simulink library "MedusaPremix"  (R2022b)
settings: Solver=VariableStepAuto  StartTime=0.0  StopTime=10.0  RelTol=1e-3
values from neighbouring files (symbols this model uses):
  PremixConfig = struct('sample_rate_in_hertz', sample_rate_in_hertz,                            'frame_size', frame_size,                            'rgain_SILENT_GAIN', rgain_SILENT_GAIN,                            'granularity', internal_granularity,                            'LR_in', LR_in, 'LR_out', LR_out,                            'CS_in', CS_in, 'CS_out', CS_out,                            'NumCenterOut' ...(+550 chars)    [MedusaPremixInit.m]
  PremixTune = MedusaPremixTuneInit(tuneFileName, headrestTuneFileName, overheadTuneFileName, MedusaParams)    [MedusaPremixInit.m]    (also in MedusaPremixTuneInit.m = load(tuneFileName))
undefined symbols (not defined in the file or in its folder): carModel, mode, MSConfig, Row
libraries: TuneVar x286, TOP x202, dspmtrx3 x146, FeaturePath x86, matrix_library x20, PooliirLib x8, Pooliir x4
(part 2 of 22)

== system MedusaPremix/Premix/Full Mixing Matrix_Center Surround ==
  Audio Channel Inputs : Inport
  RST Trigger : Inport  Port=2
  SLC Request Trigger : Inport  Port=3
  SLC In : Inport  Port=4
  SLC_NTF_check_done : Inport  Port=5
  SLC Tune In : Inport  Port=6
  Fade Request Trigger : Inport  Port=7
  Front Fade Gain : Inport  Port=8
  Back Fade Gain : Inport  Port=9
  Fade Tune In : Inport  Port=10
  Add : Sum
  Constant : Constant  OutDataTypeStr=single
  Fader Downmix : Subsystem
  FeaturePath : FeaturePath/FeaturePath  FeatureName=CS  IsGroup=off  GroupNumber=-1  DeclarePackages=off  PackageNames=mode,carModel  IsToolGroup=off  TriggerInit=[760 24 875 131]
      settings: SourceProductName=Bose Talaria
  Matrix Multiply : Product
  Premixing : Subsystem
  Subtract : Sum  Inputs=+-
  Surround Level Control : Subsystem
  Output : Outport  VectorParamsAs1DForOutWhenUnconnected=off
  SLC_NTF_done : Outport  Port=2  VectorParamsAs1DForOutWhenUnconnected=off
  wires:
  Front Fade Gain/1 -> Fader Downmix/1(Front Fade Gain)
  Add/1 -> Premixing/2(Target Gain)  "Premix Matrix"
  Premixing/1(Output) -> Output/1
  Fader Downmix/2(DownmixingMatrix) -> Add/2
  SLC Tune In/1 -> Surround Level Control/5(Tuned Inputs)
  RST Trigger/1 -> Surround Level Control/1(RST Trigger)
  Surround Level Control/2(Ramping Done) -> SLC_NTF_done/1
  Matrix Multiply/1 -> Add/1
  SLC In/1 -> Surround Level Control/3(Control Inputs)
  Fade Tune In/1 -> Fader Downmix/3(Tuned Inputs)
  Fader Downmix/1(Downmix) -> Subtract/2
  Audio Channel Inputs/1 -> Premixing/1(Audio Channel Inputs)
  SLC Request Trigger/1 -> Surround Level Control/2(SLC Request Trigger)
  SLC_NTF_check_done/1 -> Surround Level Control/4(Check Done)
  Fade Request Trigger/1 -> Fader Downmix/Trigger
  Back Fade Gain/1 -> Fader Downmix/2(Back Fade Gain)
  Constant/1 -> Subtract/1
  Subtract/1 -> Matrix Multiply/2  "No Downmix"
  Surround Level Control/1(Gain Out) -> Matrix Multiply/1

== system MedusaPremix/Premix/Full Mixing Matrix_Left ==
  Audio Channel Inputs : Inport
  RST Trigger : Inport  Port=2
  SLC Request Trigger : Inport  Port=3
  SLC In : Inport  Port=4
  SLC_NTF_check_done : Inport  Port=5
  SLC Tune In : Inport  Port=6
  Fade Request Trigger : Inport  Port=7
  Front Fade Gain : Inport  Port=8
  Back Fade Gain : Inport  Port=9
  Fade Tune In : Inport  Port=10
  Add : Sum
  Constant : Constant  OutDataTypeStr=single
  Fader Downmix : Subsystem
  FeaturePath : FeaturePath/FeaturePath  FeatureName=Left  IsGroup=off  GroupNumber=-1  DeclarePackages=off  PackageNames=mode,carModel  IsToolGroup=off  TriggerInit=[760 24 875 131]
      settings: SourceProductName=Bose Talaria
  Matrix Multiply : Product
  Premixing : Subsystem
  Subtract : Sum  Inputs=+-
  Surround Level Control : Subsystem
  Output : Outport  VectorParamsAs1DForOutWhenUnconnected=off
  SLC_NTF_done : Outport  Port=2  VectorParamsAs1DForOutWhenUnconnected=off
  wires:
  Surround Level Control/1(Gain Out) -> Matrix Multiply/1
  Front Fade Gain/1 -> Fader Downmix/1(Front Fade Gain)
  Add/1 -> Premixing/2(Target Gain)  "Premix Matrix"
  Premixing/1(Output) -> Output/1
  SLC Tune In/1 -> Surround Level Control/5(Tuned Inputs)
  Surround Level Control/2(Ramping Done) -> SLC_NTF_done/1
  Matrix Multiply/1 -> Add/1
  Fade Tune In/1 -> Fader Downmix/3(Tuned Inputs)
  Fader Downmix/1(Downmix) -> Subtract/2
  Audio Channel Inputs/1 -> Premixing/1(Audio Channel Inputs)
  SLC In/1 -> Surround Level Control/3(Control Inputs)
  SLC Request Trigger/1 -> Surround Level Control/2(SLC Request Trigger)
  SLC_NTF_check_done/1 -> Surround Level Control/4(Check Done)
  Back Fade Gain/1 -> Fader Downmix/2(Back Fade Gain)
  RST Trigger/1 -> Surround Level Control/1(RST Trigger)
  Fade Request Trigger/1 -> Fader Downmix/Trigger
  Fader Downmix/2(DownmixingMatrix) -> Add/2
  Subtract/1 -> Matrix Multiply/2  "No Downmix"
  Constant/1 -> Subtract/1

== system MedusaPremix/Premix/Full Mixing Matrix_Right ==
  Audio Channel Inputs : Inport
  RST Trigger : Inport  Port=2
  SLC Request Trigger : Inport  Port=3
  SLC In : Inport  Port=4
  SLC_NTF_check_done : Inport  Port=5
  SLC Tune In : Inport  Port=6
  Fade Request Trigger : Inport  Port=7
  Front Fade Gain : Inport  Port=8
  Back Fade Gain : Inport  Port=9
  Fade Tune In : Inport  Port=10
  Add : Sum
  Constant : Constant  OutDataTypeStr=single
  Fader Downmix : Subsystem
  FeaturePath : FeaturePath/FeaturePath  FeatureName=Right  IsGroup=off  GroupNumber=-1  DeclarePackages=off  PackageNames=mode,carModel  IsToolGroup=off  TriggerInit=[760 24 875 131]
      settings: SourceProductName=Bose Talaria
  Matrix Multiply : Product
  Premixing : Subsystem
  Subtract : Sum  Inputs=+-
  Surround Level Control : Subsystem
  Output : Outport  VectorParamsAs1DForOutWhenUnconnected=off
  SLC_NTF_done : Outport  Port=2  VectorParamsAs1DForOutWhenUnconnected=off
  wires:
  Front Fade Gain/1 -> Fader Downmix/1(Front Fade Gain)
  Add/1 -> Premixing/2(Target Gain)  "Premix Matrix"
  Premixing/1(Output) -> Output/1
  Fader Downmix/2(DownmixingMatrix) -> Add/2
  SLC Tune In/1 -> Surround Level Control/5(Tuned Inputs)
  RST Trigger/1 -> Surround Level Control/1(RST Trigger)
  Surround Level Control/2(Ramping Done) -> SLC_NTF_done/1
  Matrix Multiply/1 -> Add/1
  SLC In/1 -> Surround Level Control/3(Control Inputs)
  Fade Tune In/1 -> Fader Downmix/3(Tuned Inputs)
  Fader Downmix/1(Downmix) -> Subtract/2
  Audio Channel Inputs/1 -> Premixing/1(Audio Channel Inputs)
  SLC Request Trigger/1 -> Surround Level Control/2(SLC Request Trigger)
  SLC_NTF_check_done/1 -> Surround Level Control/4(Check Done)
  Fade Request Trigger/1 -> Fader Downmix/Trigger
  Back Fade Gain/1 -> Fader Downmix/2(Back Fade Gain)
  Constant/1 -> Subtract/1
  Subtract/1 -> Matrix Multiply/2  "No Downmix"
  Surround Level Control/1(Gain Out) -> Matrix Multiply/1

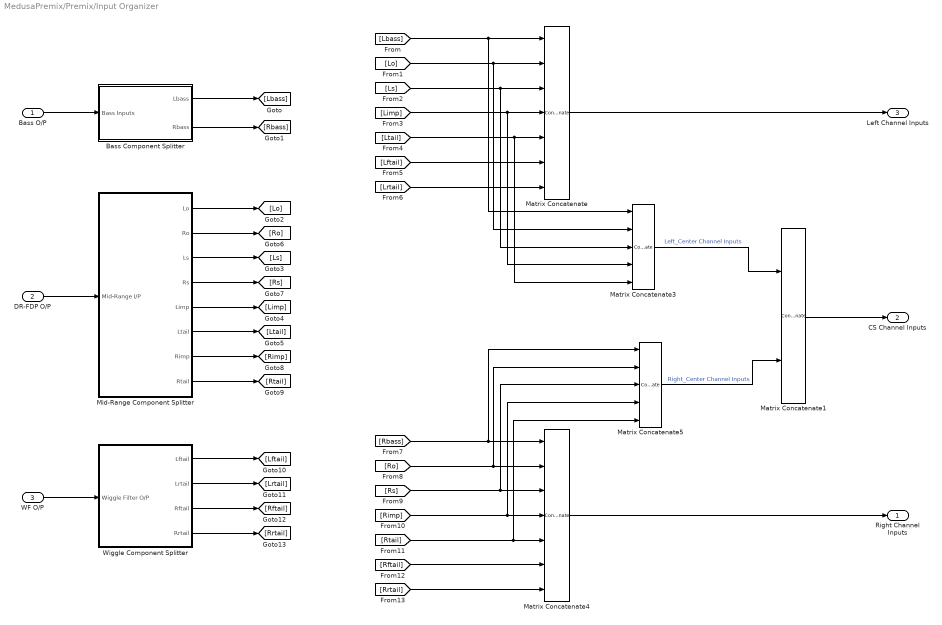
== system MedusaPremix/Premix/Input Organizer ==
  Bass O/P : Inport
  DR-FDP O/P : Inport  Port=2
  WF O/P : Inport  Port=3
  Bass Component Splitter : Subsystem
  Matrix Concatenate : Concatenate  NumInputs=7  Mode=Multidimensional array  ConcatenateDimension=2
  Matrix Concatenate1 : Concatenate  Mode=Multidimensional array  ConcatenateDimension=2
  Matrix Concatenate3 : Concatenate  NumInputs=5  Mode=Multidimensional array  ConcatenateDimension=2
  Matrix Concatenate4 : Concatenate  NumInputs=7  Mode=Multidimensional array  ConcatenateDimension=2
  Matrix Concatenate5 : Concatenate  NumInputs=5  Mode=Multidimensional array  ConcatenateDimension=2
  Mid-Range Component Splitter : Subsystem
  Wiggle Component Splitter : Subsystem
  Right Channel Inputs : Outport  VectorParamsAs1DForOutWhenUnconnected=off
  CS Channel Inputs : Outport  Port=2  VectorParamsAs1DForOutWhenUnconnected=off
  Left Channel Inputs : Outport  Port=3  VectorParamsAs1DForOutWhenUnconnected=off
  wires:
  Matrix Concatenate4/1 -> Right Channel Inputs/1
  [Ltail] -> Matrix Concatenate3/5, Matrix Concatenate/5
  Matrix Concatenate5/1 -> Matrix Concatenate1/2  "Right_Center Channel Inputs"
  [Limp] -> Matrix Concatenate3/4, Matrix Concatenate/4
  [Rimp] -> Matrix Concatenate5/4, Matrix Concatenate4/4
  [Rbass] -> Matrix Concatenate5/1, Matrix Concatenate4/1
  Matrix Concatenate1/1 -> CS Channel Inputs/1
  Wiggle Component Splitter/2(Lrtail) -> [Lrtail]
  Wiggle Component Splitter/1(Lftail) -> [Lftail]
  Bass Component Splitter/2(Rbass) -> [Rbass]
  DR-FDP O/P/1 -> Mid-Range Component Splitter/1(Mid-Range I/P)
  [Ro] -> Matrix Concatenate5/2, Matrix Concatenate4/2
  Wiggle Component Splitter/3(Rftail) -> [Rftail]
  Bass O/P/1 -> Bass Component Splitter/1(Bass Inputs)
  Matrix Concatenate/1 -> Left Channel Inputs/1
  [Lrtail] -> Matrix Concatenate/7
  [Lftail] -> Matrix Concatenate/6
  [Rs] -> Matrix Concatenate5/3, Matrix Concatenate4/3
  WF O/P/1 -> Wiggle Component Splitter/1(Wiggle Filter O/P)
  [Rtail] -> Matrix Concatenate5/5, Matrix Concatenate4/5
  [Ls] -> Matrix Concatenate3/3, Matrix Concatenate/3
  [Lbass] -> Matrix Concatenate3/1, Matrix Concatenate/1
  Matrix Concatenate3/1 -> Matrix Concatenate1/1  "Left_Center Channel Inputs"
  [Lo] -> Matrix Concatenate3/2, Matrix Concatenate/2
  Wiggle Component Splitter/4(Rrtail) -> [Rrtail]
  Mid-Range Component Splitter/1(Lo) -> [Lo]
  [Rftail] -> Matrix Concatenate4/6
  Bass Component Splitter/1(Lbass) -> [Lbass]
  [Rrtail] -> Matrix Concatenate4/7
  Mid-Range Component Splitter/2(Ro) -> [Ro]
  Mid-Range Component Splitter/3(Ls) -> [Ls]
  Mid-Range Component Splitter/4(Rs) -> [Rs]
  Mid-Range Component Splitter/5(Limp) -> [Limp]
  Mid-Range Component Splitter/6(Ltail) -> [Ltail]
  Mid-Range Component Splitter/7(Rimp) -> [Rimp]
  Mid-Range Component Splitter/8(Rtail) -> [Rtail]

== system MedusaPremix/Premix/Merge NTF_done ==
  SLC_NTF_done_Left : Inport
  SLC_NTF_done_CS : Inport  Port=2
  SLC_NTF_done_Right : Inport  Port=3
  Trigger : TriggerPort  TriggerType=function-call  VariantControl=Variant  PortDimensions=1
  AND : Logic  Inputs=3  IconShape=distinctive  AllPortsSameDT=off  OutDataTypeStr=boolean
  SLC_NTF_done : Outport  VectorParamsAs1DForOutWhenUnconnected=off
  wires:
  SLC_NTF_done_Right/1 -> AND/1
  SLC_NTF_done_CS/1 -> AND/2
  SLC_NTF_done_Left/1 -> AND/3
  AND/1 -> SLC_NTF_done/1

== system MedusaPremix/Premix/SLC Tuning ==
  Detent Level CS : Subsystem  Description="This is the premix (scalar mixing) matrix for the detent (default) level of \"surroundiness\"."
  Detent Level Left : Subsystem  Description="This is the premix (scalar mixing) matrix for the detent (default) level of \"surroundiness\"."
  Detent Level Right : Subsystem  Description="This is the premix (scalar mixing) matrix for the detent (default) level of \"surroundiness\"."
  Interpolation Method : Subsystem  Description=|
      | This controls the method used to interpolate premix coefficient matrix as the surround knob is adjusted.
      | - 0 for linear interpolation (default)
      | - 1 for db-linear interpolation
  Max Level CS : Subsystem  Description="This is the premix (scalar mixing) matrix for the maximum level of \"surroundiness\"."
  Max Level Left : Subsystem  Description="This is the premix (scalar mixing) matrix for the maximum level of \"surroundiness\"."
  Max Level Right : Subsystem  Description="This is the premix (scalar mixing) matrix for the maximum level of \"surroundiness\"."
  Min Level CS : Subsystem  Description="This is the premix (scalar mixing) matrix for the minimum level of \"surroundiness\" i.e. steroe case."
  Min Level Left : Subsystem  Description="This is the premix (scalar mixing) matrix for the minimum level of \"surroundiness\" i.e. steroe case."
  Min Level Right : Subsystem  Description="This is the premix (scalar mixing) matrix for the minimum level of \"surroundiness\" i.e. steroe case."
  Bus Element Out : Outport  VectorParamsAs1DForOutWhenUnconnected=off  PortName=SLC Tune Out  Element=Interpolation Method
  Bus Element Out1 : Outport  VectorParamsAs1DForOutWhenUnconnected=off  PortName=SLC Tune Out  Element=Min Level Left
  Bus Element Out2 : Outport  VectorParamsAs1DForOutWhenUnconnected=off  PortName=SLC Tune Out  Element=Detent Level Left
  Bus Element Out3 : Outport  VectorParamsAs1DForOutWhenUnconnected=off  PortName=SLC Tune Out  Element=Max Level Left
  Bus Element Out4 : Outport  VectorParamsAs1DForOutWhenUnconnected=off  PortName=SLC Tune Out  Element=Min Level CS
  Bus Element Out5 : Outport  VectorParamsAs1DForOutWhenUnconnected=off  PortName=SLC Tune Out  Element=Detent Level CS
  Bus Element Out6 : Outport  VectorParamsAs1DForOutWhenUnconnected=off  PortName=SLC Tune Out  Element=Max Level CS
  Bus Element Out7 : Outport  VectorParamsAs1DForOutWhenUnconnected=off  PortName=SLC Tune Out  Element=Min Level Right
  Bus Element Out8 : Outport  VectorParamsAs1DForOutWhenUnconnected=off  PortName=SLC Tune Out  Element=Detent Level Right
  Bus Element Out9 : Outport  VectorParamsAs1DForOutWhenUnconnected=off  PortName=SLC Tune Out  Element=Max Level Right
  wires:
  Interpolation Method/1(Out1) -> Bus Element Out/1
  Min Level Left/1(Out1) -> Bus Element Out1/1
  Detent Level Left/1(Out1) -> Bus Element Out2/1
  Max Level Left/1(Out1) -> Bus Element Out3/1
  Max Level CS/1(Out1) -> Bus Element Out6/1
  Min Level CS/1(Out1) -> Bus Element Out4/1
  Detent Level CS/1(Out1) -> Bus Element Out5/1
  Detent Level Right/1(Out1) -> Bus Element Out8/1
  Max Level Right/1(Out1) -> Bus Element Out9/1
  Min Level Right/1(Out1) -> Bus Element Out7/1

== system MedusaPremix/Premix51/Fade Inputs ==
  FrontGain : Inport
  BackGain : Inport  Port=2
  Abs : Abs  SaturateOnIntegerOverflow=off
  Abs1 : Abs  SaturateOnIntegerOverflow=off
  Add : Sum
  Delay : Delay  DelayLength=1  InitialCondition=0
  Delay1 : Delay  DelayLength=1  InitialCondition=0
  Fade_Trigger_Generation : MATLAB Function  TreatAsAtomicUnit=on
  Subtract1 : Sum  Inputs=-+
  Subtract2 : Sum  Inputs=-+
  triggerLeft : Outport  VectorParamsAs1DForOutWhenUnconnected=off
  triggerCS : Outport  Port=2  VectorParamsAs1DForOutWhenUnconnected=off
  triggerRight : Outport  Port=3  VectorParamsAs1DForOutWhenUnconnected=off
  FrontFadeGain : Outport  Port=4  VectorParamsAs1DForOutWhenUnconnected=off
  BackFadeGain : Outport  Port=5  VectorParamsAs1DForOutWhenUnconnected=off
  wires:
  Fade_Trigger_Generation/1(fadeTrigger_Left()) -> triggerLeft/1
  Fade_Trigger_Generation/3(fadeTrigger_Right()) -> triggerRight/1
  Add/1 -> Fade_Trigger_Generation/1(gainDifference)
  Fade_Trigger_Generation/2(fadeTrigger_CS()) -> triggerCS/1
  Delay1/1 -> Subtract2/1
  Delay/1 -> Subtract1/1
  FrontGain/1 -> Delay/1, FrontFadeGain/1, Subtract1/2
  Subtract1/1 -> Abs/1
  Subtract2/1 -> Abs1/1
  Abs/1 -> Add/1
  Abs1/1 -> Add/2
  BackGain/1 -> Delay1/1, Subtract2/2, BackFadeGain/1

== system MedusaPremix/Premix51/Fade Tuning ==
  Backward Downmix Max : Subsystem  Description=This is the fraction of downmixing that occurs when 100% fade (back) is reached.
  Backward Downmix Threshold : Subsystem  Description=This is the fraction of fade (back) at which downmixing of premix coefficients starts.
  Downmix Weights CS : Subsystem  Description=These are the mixing weights at fader extreme when downmix_max is set to 1.
  Downmix Weights Left : Subsystem  Description=These are the mixing weights at fader extreme when downmix_max is set to 1.
  Downmix Weights Right : Subsystem  Description=These are the mixing weights at fader extreme when downmix_max is set to 1.
  Forward Downmix Threshold : Subsystem  Description=This is the fraction of fade (front) at which downmixing of premix coefficients starts.
  Foward Downmix Max : Subsystem  Description=This is the fraction of downmixing that occurs when 100% fade (front) is reached.
  Bus Element Out : Outport  VectorParamsAs1DForOutWhenUnconnected=off  PortName=Fade Tune Out  Element=Forward Downmix Threshold
  Bus Element Out1 : Outport  VectorParamsAs1DForOutWhenUnconnected=off  PortName=Fade Tune Out  Element=Forward Downmix Max
  Bus Element Out2 : Outport  VectorParamsAs1DForOutWhenUnconnected=off  PortName=Fade Tune Out  Element=Backward Downmix Threshold
  Bus Element Out3 : Outport  VectorParamsAs1DForOutWhenUnconnected=off  PortName=Fade Tune Out  Element=Backward Downmix Max
  Bus Element Out4 : Outport  VectorParamsAs1DForOutWhenUnconnected=off  PortName=Fade Tune Out  Element=Downmix Weights Left
  Bus Element Out5 : Outport  VectorParamsAs1DForOutWhenUnconnected=off  PortName=Fade Tune Out  Element=Downmix Weights CS
  Bus Element Out6 : Outport  VectorParamsAs1DForOutWhenUnconnected=off  PortName=Fade Tune Out  Element=Downmix Weights Right
  wires:
  Forward Downmix Threshold/1(Out1) -> Bus Element Out/1
  Foward Downmix Max/1(Out1) -> Bus Element Out1/1
  Backward Downmix Max/1(Out1) -> Bus Element Out3/1
  Backward Downmix Threshold/1(Out1) -> Bus Element Out2/1
  Downmix Weights Left/1(Out1) -> Bus Element Out4/1
  Downmix Weights CS/1(Out1) -> Bus Element Out5/1
  Downmix Weights Right/1(Out1) -> Bus Element Out6/1

== system MedusaPremix/Premix51/Full Mixing Matrix_Center Surround ==
  Audio Channel Inputs : Inport
  RST Trigger : Inport  Port=2
  SLC Request Trigger : Inport  Port=3
  SLC In : Inport  Port=4
  SLC_NTF_check_done : Inport  Port=5
  SLC Tune In : Inport  Port=6
  Fade Request Trigger : Inport  Port=7
  Front Fade Gain : Inport  Port=8
  Back Fade Gain : Inport  Port=9
  Fade Tune In : Inport  Port=10
  Add : Sum
  Constant : Constant  OutDataTypeStr=single
  Fader Downmix : Subsystem
  FeaturePath : FeaturePath/FeaturePath  FeatureName=CS  IsGroup=off  GroupNumber=-1  DeclarePackages=off  PackageNames=mode,carModel  IsToolGroup=off  TriggerInit=[760 24 875 131]
      settings: SourceProductName=Bose Talaria
  Matrix Multiply : Product
  Premixing : Subsystem
  Subtract : Sum  Inputs=+-
  Surround Level Control : Subsystem
  Output : Outport  VectorParamsAs1DForOutWhenUnconnected=off
  SLC_NTF_done : Outport  Port=2  VectorParamsAs1DForOutWhenUnconnected=off
  wires:
  Surround Level Control/1(Gain Out) -> Matrix Multiply/1
  Front Fade Gain/1 -> Fader Downmix/1(Front Fade Gain)
  Add/1 -> Premixing/2(Target Gain)  "Premix Matrix"
  Premixing/1(Output) -> Output/1
  Fader Downmix/2(DownmixingMatrix) -> Add/2
  SLC Tune In/1 -> Surround Level Control/5(Tuned Inputs)
  RST Trigger/1 -> Surround Level Control/1(RST Trigger)
  Surround Level Control/2(Ramping Done) -> SLC_NTF_done/1
  Matrix Multiply/1 -> Add/1
  SLC In/1 -> Surround Level Control/3(Control Inputs)
  Fade Tune In/1 -> Fader Downmix/3(Tuned Inputs)
  Fader Downmix/1(Downmix) -> Subtract/2
  Audio Channel Inputs/1 -> Premixing/1(Audio Channel Inputs)
  SLC Request Trigger/1 -> Surround Level Control/2(SLC Request Trigger)
  SLC_NTF_check_done/1 -> Surround Level Control/4(Check Done)
  Fade Request Trigger/1 -> Fader Downmix/Trigger
  Back Fade Gain/1 -> Fader Downmix/2(Back Fade Gain)
  Constant/1 -> Subtract/1
  Subtract/1 -> Matrix Multiply/2  "No Downmix"

== system MedusaPremix/Premix51/Full Mixing Matrix_Left ==
  Audio Channel Inputs : Inport
  RST Trigger : Inport  Port=2
  SLC Request Trigger : Inport  Port=3
  SLC In : Inport  Port=4
  SLC_NTF_check_done : Inport  Port=5
  SLC Tune In : Inport  Port=6
  Fade Request Trigger : Inport  Port=7
  Front Fade Gain : Inport  Port=8
  Back Fade Gain : Inport  Port=9
  Fade Tune In : Inport  Port=10
  Add : Sum
  Constant : Constant  OutDataTypeStr=single
  Fader Downmix : Subsystem
  FeaturePath : FeaturePath/FeaturePath  FeatureName=Left  IsGroup=off  GroupNumber=-1  DeclarePackages=off  PackageNames=mode,carModel  IsToolGroup=off  TriggerInit=[760 24 875 131]
      settings: SourceProductName=Bose Talaria
  Matrix Multiply : Product
  Premixing : Subsystem
  Subtract : Sum  Inputs=+-
  Surround Level Control : Subsystem
  Output : Outport  VectorParamsAs1DForOutWhenUnconnected=off
  SLC_NTF_done : Outport  Port=2  VectorParamsAs1DForOutWhenUnconnected=off
  wires:
  Surround Level Control/1(Gain Out) -> Matrix Multiply/1
  Front Fade Gain/1 -> Fader Downmix/1(Front Fade Gain)
  Add/1 -> Premixing/2(Target Gain)  "Premix Matrix"
  Premixing/1(Output) -> Output/1
  SLC Tune In/1 -> Surround Level Control/5(Tuned Inputs)
  Surround Level Control/2(Ramping Done) -> SLC_NTF_done/1
  Matrix Multiply/1 -> Add/1
  Fade Tune In/1 -> Fader Downmix/3(Tuned Inputs)
  Fader Downmix/1(Downmix) -> Subtract/2
  Audio Channel Inputs/1 -> Premixing/1(Audio Channel Inputs)
  SLC In/1 -> Surround Level Control/3(Control Inputs)
  SLC Request Trigger/1 -> Surround Level Control/2(SLC Request Trigger)
  SLC_NTF_check_done/1 -> Surround Level Control/4(Check Done)
  Back Fade Gain/1 -> Fader Downmix/2(Back Fade Gain)
  RST Trigger/1 -> Surround Level Control/1(RST Trigger)
  Fade Request Trigger/1 -> Fader Downmix/Trigger
  Fader Downmix/2(DownmixingMatrix) -> Add/2
  Subtract/1 -> Matrix Multiply/2  "No Downmix"
  Constant/1 -> Subtract/1

== system MedusaPremix/Premix51/Full Mixing Matrix_Right ==
  Audio Channel Inputs : Inport
  RST Trigger : Inport  Port=2
  SLC Request Trigger : Inport  Port=3
  SLC In : Inport  Port=4
  SLC_NTF_check_done : Inport  Port=5
  SLC Tune In : Inport  Port=6
  Fade Request Trigger : Inport  Port=7
  Front Fade Gain : Inport  Port=8
  Back Fade Gain : Inport  Port=9
  Fade Tune In : Inport  Port=10
  Add : Sum
  Constant : Constant  OutDataTypeStr=single
  Fader Downmix : Subsystem
  FeaturePath : FeaturePath/FeaturePath  FeatureName=Right  IsGroup=off  GroupNumber=-1  DeclarePackages=off  PackageNames=mode,carModel  IsToolGroup=off  TriggerInit=[760 24 875 131]
      settings: SourceProductName=Bose Talaria
  Matrix Multiply : Product
  Premixing : Subsystem
  Subtract : Sum  Inputs=+-
  Surround Level Control : Subsystem
  Output : Outport  VectorParamsAs1DForOutWhenUnconnected=off
  SLC_NTF_done : Outport  Port=2  VectorParamsAs1DForOutWhenUnconnected=off
  wires:
  Surround Level Control/1(Gain Out) -> Matrix Multiply/1
  Front Fade Gain/1 -> Fader Downmix/1(Front Fade Gain)
  Add/1 -> Premixing/2(Target Gain)  "Premix Matrix"
  Premixing/1(Output) -> Output/1
  Fader Downmix/2(DownmixingMatrix) -> Add/2
  SLC Tune In/1 -> Surround Level Control/5(Tuned Inputs)
  RST Trigger/1 -> Surround Level Control/1(RST Trigger)
  Surround Level Control/2(Ramping Done) -> SLC_NTF_done/1
  Matrix Multiply/1 -> Add/1
  SLC In/1 -> Surround Level Control/3(Control Inputs)
  Fade Tune In/1 -> Fader Downmix/3(Tuned Inputs)
  Fader Downmix/1(Downmix) -> Subtract/2
  Audio Channel Inputs/1 -> Premixing/1(Audio Channel Inputs)
  SLC Request Trigger/1 -> Surround Level Control/2(SLC Request Trigger)
  SLC_NTF_check_done/1 -> Surround Level Control/4(Check Done)
  Fade Request Trigger/1 -> Fader Downmix/Trigger
  Back Fade Gain/1 -> Fader Downmix/2(Back Fade Gain)
  Constant/1 -> Subtract/1
  Subtract/1 -> Matrix Multiply/2  "No Downmix"

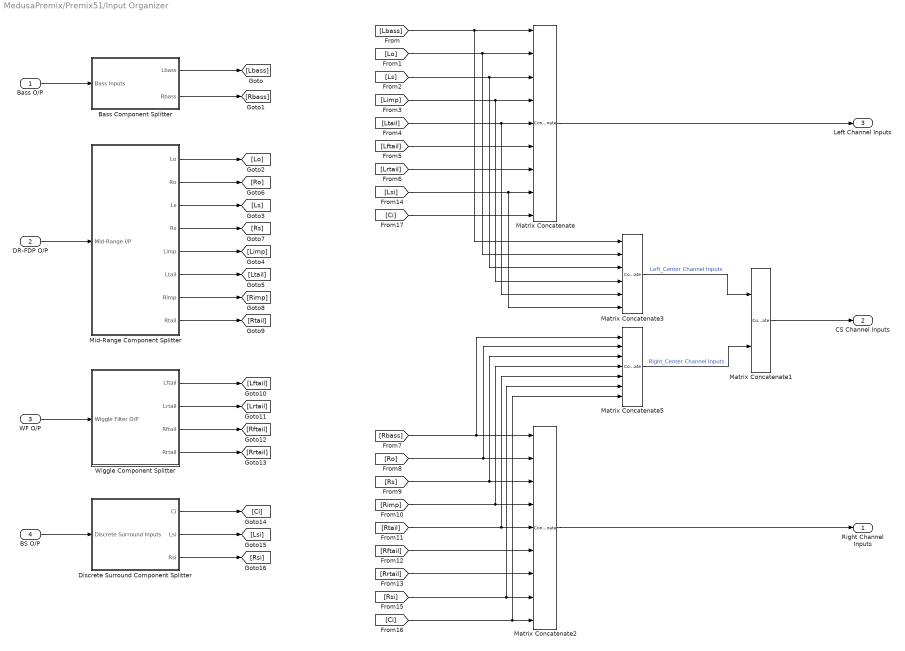
== system MedusaPremix/Premix51/Input Organizer ==
  Bass O/P : Inport
  DR-FDP O/P : Inport  Port=2
  WF O/P : Inport  Port=3
  BS O/P : Inport  Port=4
  Bass Component Splitter : Subsystem
  Discrete Surround Component Splitter : Subsystem
  Matrix Concatenate : Concatenate  NumInputs=9  Mode=Multidimensional array  ConcatenateDimension=2
  Matrix Concatenate1 : Concatenate  Mode=Multidimensional array  ConcatenateDimension=2
  Matrix Concatenate2 : Concatenate  NumInputs=9  Mode=Multidimensional array  ConcatenateDimension=2
  Matrix Concatenate3 : Concatenate  NumInputs=6  Mode=Multidimensional array  ConcatenateDimension=2
  Matrix Concatenate5 : Concatenate  NumInputs=7  Mode=Multidimensional array  ConcatenateDimension=2
  Mid-Range Component Splitter : Subsystem
  Wiggle Component Splitter : Subsystem
  Right Channel Inputs : Outport  VectorParamsAs1DForOutWhenUnconnected=off
  CS Channel Inputs : Outport  Port=2  VectorParamsAs1DForOutWhenUnconnected=off
  Left Channel Inputs : Outport  Port=3  VectorParamsAs1DForOutWhenUnconnected=off
  wires:
  Matrix Concatenate2/1 -> Right Channel Inputs/1
  [Ltail] -> Matrix Concatenate/5, Matrix Concatenate3/5
  Matrix Concatenate5/1 -> Matrix Concatenate1/2  "Right_Center Channel Inputs"
  [Limp] -> Matrix Concatenate/4, Matrix Concatenate3/4
  [Rimp] -> Matrix Concatenate2/4, Matrix Concatenate5/4
  [Rbass] -> Matrix Concatenate2/1, Matrix Concatenate5/1
  Matrix Concatenate1/1 -> CS Channel Inputs/1
  Wiggle Component Splitter/2(Lrtail) -> [Lrtail]
  Wiggle Component Splitter/1(Lftail) -> [Lftail]
  Bass Component Splitter/2(Rbass) -> [Rbass]
  DR-FDP O/P/1 -> Mid-Range Component Splitter/1(Mid-Range I/P)
  [Ro] -> Matrix Concatenate2/2, Matrix Concatenate5/2
  Wiggle Component Splitter/3(Rftail) -> [Rftail]
  Bass O/P/1 -> Bass Component Splitter/1(Bass Inputs)
  Matrix Concatenate/1 -> Left Channel Inputs/1
  [Lrtail] -> Matrix Concatenate/7
  [Lftail] -> Matrix Concatenate/6
  [Rs] -> Matrix Concatenate2/3, Matrix Concatenate5/3
  WF O/P/1 -> Wiggle Component Splitter/1(Wiggle Filter O/P)
  [Rtail] -> Matrix Concatenate2/5, Matrix Concatenate5/5
  [Ls] -> Matrix Concatenate/3, Matrix Concatenate3/3
  [Lbass] -> Matrix Concatenate/1, Matrix Concatenate3/1
  Matrix Concatenate3/1 -> Matrix Concatenate1/1  "Left_Center Channel Inputs"
  [Lo] -> Matrix Concatenate/2, Matrix Concatenate3/2
  Wiggle Component Splitter/4(Rrtail) -> [Rrtail]
  Mid-Range Component Splitter/1(Lo) -> [Lo]
  [Rftail] -> Matrix Concatenate2/6
  Bass Component Splitter/1(Lbass) -> [Lbass]
  [Rrtail] -> Matrix Concatenate2/7
  Mid-Range Component Splitter/2(Ro) -> [Ro]
  Mid-Range Component Splitter/3(Ls) -> [Ls]
  Mid-Range Component Splitter/4(Rs) -> [Rs]
  Mid-Range Component Splitter/5(Limp) -> [Limp]
  Mid-Range Component Splitter/6(Ltail) -> [Ltail]
  Mid-Range Component Splitter/7(Rimp) -> [Rimp]
  Mid-Range Component Splitter/8(Rtail) -> [Rtail]
  BS O/P/1 -> Discrete Surround Component Splitter/1(Discrete Surround Inputs)
  Discrete Surround Component Splitter/2(Lsi) -> [Lsi]
  Discrete Surround Component Splitter/1(Ci) -> [Ci]
  Discrete Surround Component Splitter/3(Rsi) -> [Rsi]
  [Lsi] -> Matrix Concatenate/8, Matrix Concatenate3/6
  [Rsi] -> Matrix Concatenate2/8, Matrix Concatenate5/6
  [Ci] -> Matrix Concatenate5/7, Matrix Concatenate2/9
  [Ci] -> Matrix Concatenate/9

== system MedusaPremix/Premix51/Merge NTF_done ==
  SLC_NTF_done_Left : Inport
  SLC_NTF_done_CS : Inport  Port=2
  SLC_NTF_done_Right : Inport  Port=3
  Trigger : TriggerPort  TriggerType=function-call  VariantControl=Variant  PortDimensions=1
  AND : Logic  Inputs=3  IconShape=distinctive  AllPortsSameDT=off  OutDataTypeStr=boolean
  SLC_NTF_done : Outport  VectorParamsAs1DForOutWhenUnconnected=off
  wires:
  SLC_NTF_done_Right/1 -> AND/1
  SLC_NTF_done_CS/1 -> AND/2
  SLC_NTF_done_Left/1 -> AND/3
  AND/1 -> SLC_NTF_done/1

== system MedusaPremix/Premix51/SLC Tuning ==
  Detent Level CS : Subsystem  Description="This is the premix (scalar mixing) matrix for the detent (default) level of \"surroundiness\"."
  Detent Level Left : Subsystem  Description="This is the premix (scalar mixing) matrix for the detent (default) level of \"surroundiness\"."
  Detent Level Right : Subsystem  Description="This is the premix (scalar mixing) matrix for the detent (default) level of \"surroundiness\"."
  Interpolation Method : Subsystem  Description=|
      | This controls the method used to interpolate premix coefficient matrix as the surround knob is adjusted.
      | - 0 for linear interpolation (default)
      | - 1 for db-linear interpolation
  Max Level CS : Subsystem  Description="This is the premix (scalar mixing) matrix for the maximum level of \"surroundiness\"."
  Max Level Left : Subsystem  Description="This is the premix (scalar mixing) matrix for the maximum level of \"surroundiness\"."
  Max Level Right : Subsystem  Description="This is the premix (scalar mixing) matrix for the maximum level of \"surroundiness\"."
  Min Level CS : Subsystem  Description="This is the premix (scalar mixing) matrix for the minimum level of \"surroundiness\" i.e. steroe case."
  Min Level Left : Subsystem  Description="This is the premix (scalar mixing) matrix for the minimum level of \"surroundiness\" i.e. steroe case."
  Min Level Right : Subsystem  Description="This is the premix (scalar mixing) matrix for the minimum level of \"surroundiness\" i.e. steroe case."
  Bus Element Out : Outport  VectorParamsAs1DForOutWhenUnconnected=off  PortName=SLC Tune Out  Element=Interpolation Method
  Bus Element Out1 : Outport  VectorParamsAs1DForOutWhenUnconnected=off  PortName=SLC Tune Out  Element=Min Level Left
  Bus Element Out2 : Outport  VectorParamsAs1DForOutWhenUnconnected=off  PortName=SLC Tune Out  Element=Detent Level Left
  Bus Element Out3 : Outport  VectorParamsAs1DForOutWhenUnconnected=off  PortName=SLC Tune Out  Element=Max Level Left
  Bus Element Out4 : Outport  VectorParamsAs1DForOutWhenUnconnected=off  PortName=SLC Tune Out  Element=Min Level CS
  Bus Element Out5 : Outport  VectorParamsAs1DForOutWhenUnconnected=off  PortName=SLC Tune Out  Element=Detent Level CS
  Bus Element Out6 : Outport  VectorParamsAs1DForOutWhenUnconnected=off  PortName=SLC Tune Out  Element=Max Level CS
  Bus Element Out7 : Outport  VectorParamsAs1DForOutWhenUnconnected=off  PortName=SLC Tune Out  Element=Min Level Right
  Bus Element Out8 : Outport  VectorParamsAs1DForOutWhenUnconnected=off  PortName=SLC Tune Out  Element=Detent Level Right
  Bus Element Out9 : Outport  VectorParamsAs1DForOutWhenUnconnected=off  PortName=SLC Tune Out  Element=Max Level Right
  wires:
  Interpolation Method/1(Out1) -> Bus Element Out/1
  Min Level Left/1(Out1) -> Bus Element Out1/1
  Detent Level Left/1(Out1) -> Bus Element Out2/1
  Max Level Left/1(Out1) -> Bus Element Out3/1
  Max Level CS/1(Out1) -> Bus Element Out6/1
  Min Level CS/1(Out1) -> Bus Element Out4/1
  Detent Level CS/1(Out1) -> Bus Element Out5/1
  Detent Level Right/1(Out1) -> Bus Element Out8/1
  Max Level Right/1(Out1) -> Bus Element Out9/1
  Min Level Right/1(Out1) -> Bus Element Out7/1

== system MedusaPremix/Premix51WithMonoSurround/CS Processing ==
  COut : Inport
  ChanIn : Inport  Port=2
  MixCoeff : Inport  Port=3
  Constant : Constant  Value=MedusaPremixConfig.NumSurroundOut  SampleTime=-1
  Mono-Surround : Subsystem
  Selective Concatenation : MATLAB Function  TreatAsAtomicUnit=on
  CSOut : Outport  VectorParamsAs1DForOutWhenUnconnected=off
  wires:
  ChanIn/1 -> Mono-Surround/1(ChanIn)
  Mono-Surround/1(S) -> Selective Concatenation/2(S)
  COut/1 -> Selective Concatenation/1(COut)
  MixCoeff/1 -> Mono-Surround/2(MixCoeff)
  Selective Concatenation/1(CSOut) -> CSOut/1
  Constant/1 -> Mono-Surround/Enable

== system MedusaPremix/Premix51WithMonoSurround/Fade Inputs ==
  FrontGain : Inport
  BackGain : Inport  Port=2
  Abs : Abs  SaturateOnIntegerOverflow=off
  Abs1 : Abs  SaturateOnIntegerOverflow=off
  Add : Sum
  Delay : Delay  DelayLength=1  InitialCondition=0
  Delay1 : Delay  DelayLength=1  InitialCondition=0
  Fade_Trigger_Generation : MATLAB Function  TreatAsAtomicUnit=on
  Subtract1 : Sum  Inputs=-+
  Subtract2 : Sum  Inputs=-+
  triggerLeft : Outport  VectorParamsAs1DForOutWhenUnconnected=off
  triggerCS : Outport  Port=2  VectorParamsAs1DForOutWhenUnconnected=off
  triggerRight : Outport  Port=3  VectorParamsAs1DForOutWhenUnconnected=off
  FrontFadeGain : Outport  Port=4  VectorParamsAs1DForOutWhenUnconnected=off
  BackFadeGain : Outport  Port=5  VectorParamsAs1DForOutWhenUnconnected=off
  wires:
  Fade_Trigger_Generation/1(fadeTrigger_Left()) -> triggerLeft/1
  Fade_Trigger_Generation/3(fadeTrigger_Right()) -> triggerRight/1
  Add/1 -> Fade_Trigger_Generation/1(gainDifference)
  Fade_Trigger_Generation/2(fadeTrigger_CS()) -> triggerCS/1
  Delay1/1 -> Subtract2/1
  Delay/1 -> Subtract1/1
  FrontGain/1 -> Delay/1, FrontFadeGain/1, Subtract1/2
  Subtract1/1 -> Abs/1
  Subtract2/1 -> Abs1/1
  Abs/1 -> Add/1
  Abs1/1 -> Add/2
  BackGain/1 -> Delay1/1, Subtract2/2, BackFadeGain/1

== system MedusaPremix/Premix51WithMonoSurround/Fade Tuning ==
  Backward Downmix Max : Subsystem  Description=This is the fraction of downmixing that occurs when 100% fade (back) is reached.
  Backward Downmix Threshold : Subsystem  Description=This is the fraction of fade (back) at which downmixing of premix coefficients starts.
  Downmix Weights CS : Subsystem  Description=These are the mixing weights at fader extreme when downmix_max is set to 1.
  Downmix Weights Left : Subsystem  Description=These are the mixing weights at fader extreme when downmix_max is set to 1.
  Downmix Weights Right : Subsystem  Description=These are the mixing weights at fader extreme when downmix_max is set to 1.
  Forward Downmix Threshold : Subsystem  Description=This is the fraction of fade (front) at which downmixing of premix coefficients starts.
  Foward Downmix Max : Subsystem  Description=This is the fraction of downmixing that occurs when 100% fade (front) is reached.
  Bus Element Out : Outport  VectorParamsAs1DForOutWhenUnconnected=off  PortName=Fade Tune Out  Element=Forward Downmix Threshold
  Bus Element Out1 : Outport  VectorParamsAs1DForOutWhenUnconnected=off  PortName=Fade Tune Out  Element=Forward Downmix Max
  Bus Element Out2 : Outport  VectorParamsAs1DForOutWhenUnconnected=off  PortName=Fade Tune Out  Element=Backward Downmix Threshold
  Bus Element Out3 : Outport  VectorParamsAs1DForOutWhenUnconnected=off  PortName=Fade Tune Out  Element=Backward Downmix Max
  Bus Element Out4 : Outport  VectorParamsAs1DForOutWhenUnconnected=off  PortName=Fade Tune Out  Element=Downmix Weights Left
  Bus Element Out5 : Outport  VectorParamsAs1DForOutWhenUnconnected=off  PortName=Fade Tune Out  Element=Downmix Weights CS
  Bus Element Out6 : Outport  VectorParamsAs1DForOutWhenUnconnected=off  PortName=Fade Tune Out  Element=Downmix Weights Right
  wires:
  Forward Downmix Threshold/1(Out1) -> Bus Element Out/1
  Foward Downmix Max/1(Out1) -> Bus Element Out1/1
  Backward Downmix Max/1(Out1) -> Bus Element Out3/1
  Backward Downmix Threshold/1(Out1) -> Bus Element Out2/1
  Downmix Weights Left/1(Out1) -> Bus Element Out4/1
  Downmix Weights CS/1(Out1) -> Bus Element Out5/1
  Downmix Weights Right/1(Out1) -> Bus Element Out6/1

== system MedusaPremix/Premix51WithMonoSurround/Full Mixing Matrix_Center Surround ==
  Audio Channel Inputs : Inport
  RST Trigger : Inport  Port=2
  SLC Request Trigger : Inport  Port=3
  SLC In : Inport  Port=4
  SLC_NTF_check_done : Inport  Port=5
  SLC Tune In : Inport  Port=6
  Fade Request Trigger : Inport  Port=7
  Front Fade Gain : Inport  Port=8
  Back Fade Gain : Inport  Port=9
  Fade Tune In : Inport  Port=10
  Add : Sum
  Constant : Constant  OutDataTypeStr=single
  Fader Downmix : Subsystem
  FeaturePath : FeaturePath/FeaturePath  FeatureName=CS  IsGroup=off  GroupNumber=-1  DeclarePackages=off  PackageNames=mode,carModel  IsToolGroup=off  TriggerInit=[760 24 875 131]
      settings: SourceProductName=Bose Talaria
  Matrix Multiply : Product
  Premixing : Subsystem
  Submatrix : dspmtrx3/Submatrix  RowSpan=One row  RowStartMode=Last  RowStartIndex=1  RowEndMode=Last  RowEndIndex=1  ColSpan=All columns  ColStartMode=First  ColStartIndex=1  ColEndMode=Last  ColEndIndex=1
  Submatrix1 : dspmtrx3/Submatrix  RowSpan=Range of rows  RowStartMode=First  RowStartIndex=1  RowEndMode=Index  RowEndIndex=MedusaPremixConfig.NumCenterOut  ColSpan=All columns  ColStartMode=First  ColStartIndex=1  ColEndMode=Last  ColEndIndex=1
  Subtract : Sum  Inputs=+-
  Surround Level Control : Subsystem
  Output : Outport  VectorParamsAs1DForOutWhenUnconnected=off
  MS Mixing Gains : Outport  Port=2  VectorParamsAs1DForOutWhenUnconnected=off
  SLC_NTF_done : Outport  Port=3  VectorParamsAs1DForOutWhenUnconnected=off
  wires:
  Surround Level Control/1(Gain Out) -> Matrix Multiply/1
  Front Fade Gain/1 -> Fader Downmix/1(Front Fade Gain)
  Premixing/1(Output) -> Output/1
  Fader Downmix/2(DownmixingMatrix) -> Add/2
  SLC Tune In/1 -> Surround Level Control/5(Tuned Inputs)
  RST Trigger/1 -> Surround Level Control/1(RST Trigger)
  Surround Level Control/2(Ramping Done) -> SLC_NTF_done/1
  Matrix Multiply/1 -> Add/1
  SLC In/1 -> Surround Level Control/3(Control Inputs)
  Fade Tune In/1 -> Fader Downmix/3(Tuned Inputs)
  Fader Downmix/1(Downmix) -> Subtract/2
  Audio Channel Inputs/1 -> Premixing/1(Audio Channel Inputs)
  SLC Request Trigger/1 -> Surround Level Control/2(SLC Request Trigger)
  SLC_NTF_check_done/1 -> Surround Level Control/4(Check Done)
  Fade Request Trigger/1 -> Fader Downmix/Trigger
  Back Fade Gain/1 -> Fader Downmix/2(Back Fade Gain)
  Constant/1 -> Subtract/1
  Subtract/1 -> Matrix Multiply/2  "No Downmix"
  Submatrix/1 -> MS Mixing Gains/1
  Add/1 -> Submatrix1/1, Submatrix/1  "Premix Matrix"
  Submatrix1/1 -> Premixing/2(Target Gain)

== system MedusaPremix/Premix51WithMonoSurround/Full Mixing Matrix_Left ==
  Audio Channel Inputs : Inport
  RST Trigger : Inport  Port=2
  SLC Request Trigger : Inport  Port=3
  SLC In : Inport  Port=4
  SLC_NTF_check_done : Inport  Port=5
  SLC Tune In : Inport  Port=6
  Fade Request Trigger : Inport  Port=7
  Front Fade Gain : Inport  Port=8
  Back Fade Gain : Inport  Port=9
  Fade Tune In : Inport  Port=10
  Add : Sum
  Constant : Constant  OutDataTypeStr=single
  Fader Downmix : Subsystem
  FeaturePath : FeaturePath/FeaturePath  FeatureName=Left  IsGroup=off  GroupNumber=-1  DeclarePackages=off  PackageNames=mode,carModel  IsToolGroup=off  TriggerInit=[760 24 875 131]
      settings: SourceProductName=Bose Talaria
  Matrix Multiply : Product
  Premixing : Subsystem
  Subtract : Sum  Inputs=+-
  Surround Level Control : Subsystem
  Output : Outport  VectorParamsAs1DForOutWhenUnconnected=off
  SLC_NTF_done : Outport  Port=2  VectorParamsAs1DForOutWhenUnconnected=off
  wires:
  Surround Level Control/1(Gain Out) -> Matrix Multiply/1
  Front Fade Gain/1 -> Fader Downmix/1(Front Fade Gain)
  Add/1 -> Premixing/2(Target Gain)  "Premix Matrix"
  Premixing/1(Output) -> Output/1
  SLC Tune In/1 -> Surround Level Control/5(Tuned Inputs)
  Surround Level Control/2(Ramping Done) -> SLC_NTF_done/1
  Matrix Multiply/1 -> Add/1
  Fade Tune In/1 -> Fader Downmix/3(Tuned Inputs)
  Fader Downmix/1(Downmix) -> Subtract/2
  Audio Channel Inputs/1 -> Premixing/1(Audio Channel Inputs)
  SLC In/1 -> Surround Level Control/3(Control Inputs)
  SLC Request Trigger/1 -> Surround Level Control/2(SLC Request Trigger)
  SLC_NTF_check_done/1 -> Surround Level Control/4(Check Done)
  Back Fade Gain/1 -> Fader Downmix/2(Back Fade Gain)
  RST Trigger/1 -> Surround Level Control/1(RST Trigger)
  Fade Request Trigger/1 -> Fader Downmix/Trigger
  Fader Downmix/2(DownmixingMatrix) -> Add/2
  Subtract/1 -> Matrix Multiply/2  "No Downmix"
  Constant/1 -> Subtract/1

== system MedusaPremix/Premix51WithMonoSurround/Full Mixing Matrix_Right ==
  Audio Channel Inputs : Inport
  RST Trigger : Inport  Port=2
  SLC Request Trigger : Inport  Port=3
  SLC In : Inport  Port=4
  SLC_NTF_check_done : Inport  Port=5
  SLC Tune In : Inport  Port=6
  Fade Request Trigger : Inport  Port=7
  Front Fade Gain : Inport  Port=8
  Back Fade Gain : Inport  Port=9
  Fade Tune In : Inport  Port=10
  Add : Sum
  Constant : Constant  OutDataTypeStr=single
  Fader Downmix : Subsystem
  FeaturePath : FeaturePath/FeaturePath  FeatureName=Right  IsGroup=off  GroupNumber=-1  DeclarePackages=off  PackageNames=mode,carModel  IsToolGroup=off  TriggerInit=[760 24 875 131]
      settings: SourceProductName=Bose Talaria
  Matrix Multiply : Product
  Premixing : Subsystem
  Subtract : Sum  Inputs=+-
  Surround Level Control : Subsystem
  Output : Outport  VectorParamsAs1DForOutWhenUnconnected=off
  SLC_NTF_done : Outport  Port=2  VectorParamsAs1DForOutWhenUnconnected=off
  wires:
  Surround Level Control/1(Gain Out) -> Matrix Multiply/1
  Front Fade Gain/1 -> Fader Downmix/1(Front Fade Gain)
  Add/1 -> Premixing/2(Target Gain)  "Premix Matrix"
  Premixing/1(Output) -> Output/1
  Fader Downmix/2(DownmixingMatrix) -> Add/2
  SLC Tune In/1 -> Surround Level Control/5(Tuned Inputs)
  RST Trigger/1 -> Surround Level Control/1(RST Trigger)
  Surround Level Control/2(Ramping Done) -> SLC_NTF_done/1
  Matrix Multiply/1 -> Add/1
  SLC In/1 -> Surround Level Control/3(Control Inputs)
  Fade Tune In/1 -> Fader Downmix/3(Tuned Inputs)
  Fader Downmix/1(Downmix) -> Subtract/2
  Audio Channel Inputs/1 -> Premixing/1(Audio Channel Inputs)
  SLC Request Trigger/1 -> Surround Level Control/2(SLC Request Trigger)
  SLC_NTF_check_done/1 -> Surround Level Control/4(Check Done)
  Fade Request Trigger/1 -> Fader Downmix/Trigger
  Back Fade Gain/1 -> Fader Downmix/2(Back Fade Gain)
  Constant/1 -> Subtract/1
  Subtract/1 -> Matrix Multiply/2  "No Downmix"

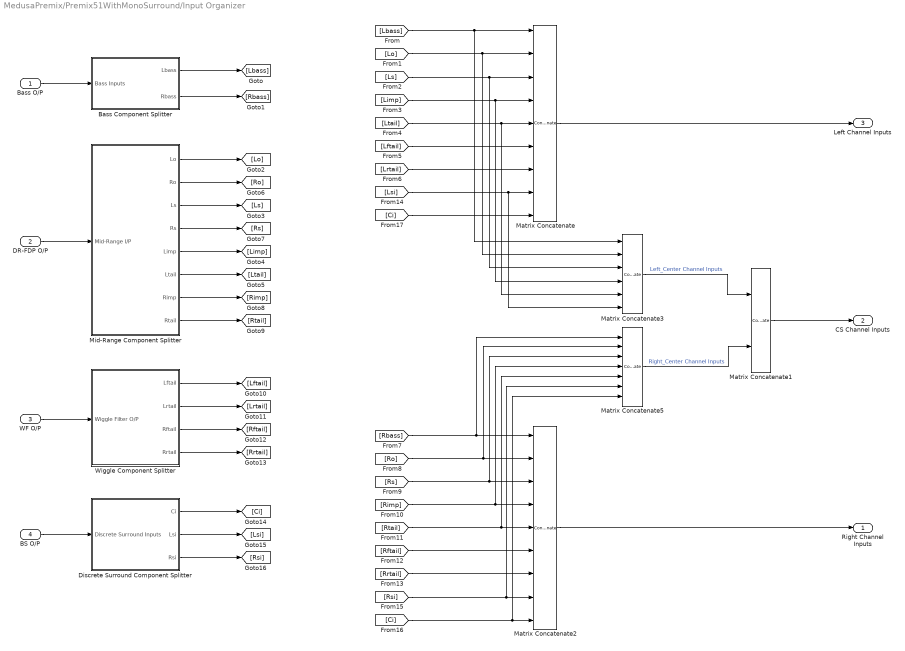
== system MedusaPremix/Premix51WithMonoSurround/Input Organizer ==
  Bass O/P : Inport
  DR-FDP O/P : Inport  Port=2
  WF O/P : Inport  Port=3
  BS O/P : Inport  Port=4
  Bass Component Splitter : Subsystem
  Discrete Surround Component Splitter : Subsystem
  Matrix Concatenate : Concatenate  NumInputs=9  Mode=Multidimensional array  ConcatenateDimension=2
  Matrix Concatenate1 : Concatenate  Mode=Multidimensional array  ConcatenateDimension=2
  Matrix Concatenate2 : Concatenate  NumInputs=9  Mode=Multidimensional array  ConcatenateDimension=2
  Matrix Concatenate3 : Concatenate  NumInputs=6  Mode=Multidimensional array  ConcatenateDimension=2
  Matrix Concatenate5 : Concatenate  NumInputs=7  Mode=Multidimensional array  ConcatenateDimension=2
  Mid-Range Component Splitter : Subsystem
  Wiggle Component Splitter : Subsystem
  Right Channel Inputs : Outport  VectorParamsAs1DForOutWhenUnconnected=off
  CS Channel Inputs : Outport  Port=2  VectorParamsAs1DForOutWhenUnconnected=off
  Left Channel Inputs : Outport  Port=3  VectorParamsAs1DForOutWhenUnconnected=off
  wires:
  Matrix Concatenate2/1 -> Right Channel Inputs/1
  [Ltail] -> Matrix Concatenate/5, Matrix Concatenate3/5
  Matrix Concatenate5/1 -> Matrix Concatenate1/2  "Right_Center Channel Inputs"
  [Limp] -> Matrix Concatenate/4, Matrix Concatenate3/4
  [Rimp] -> Matrix Concatenate2/4, Matrix Concatenate5/4
  [Rbass] -> Matrix Concatenate2/1, Matrix Concatenate5/1
  Matrix Concatenate1/1 -> CS Channel Inputs/1
  Wiggle Component Splitter/2(Lrtail) -> [Lrtail]
  Wiggle Component Splitter/1(Lftail) -> [Lftail]
  Bass Component Splitter/2(Rbass) -> [Rbass]
  DR-FDP O/P/1 -> Mid-Range Component Splitter/1(Mid-Range I/P)
  [Ro] -> Matrix Concatenate2/2, Matrix Concatenate5/2
  Wiggle Component Splitter/3(Rftail) -> [Rftail]
  Bass O/P/1 -> Bass Component Splitter/1(Bass Inputs)
  Matrix Concatenate/1 -> Left Channel Inputs/1
  [Lrtail] -> Matrix Concatenate/7
  [Lftail] -> Matrix Concatenate/6
  [Rs] -> Matrix Concatenate2/3, Matrix Concatenate5/3
  WF O/P/1 -> Wiggle Component Splitter/1(Wiggle Filter O/P)
  [Rtail] -> Matrix Concatenate2/5, Matrix Concatenate5/5
  [Ls] -> Matrix Concatenate/3, Matrix Concatenate3/3
  [Lbass] -> Matrix Concatenate/1, Matrix Concatenate3/1
  Matrix Concatenate3/1 -> Matrix Concatenate1/1  "Left_Center Channel Inputs"
  [Lo] -> Matrix Concatenate/2, Matrix Concatenate3/2
  Wiggle Component Splitter/4(Rrtail) -> [Rrtail]
  Mid-Range Component Splitter/1(Lo) -> [Lo]
  [Rftail] -> Matrix Concatenate2/6
  Bass Component Splitter/1(Lbass) -> [Lbass]
  [Rrtail] -> Matrix Concatenate2/7
  Mid-Range Component Splitter/2(Ro) -> [Ro]
  Mid-Range Component Splitter/3(Ls) -> [Ls]
  Mid-Range Component Splitter/4(Rs) -> [Rs]
  Mid-Range Component Splitter/5(Limp) -> [Limp]
  Mid-Range Component Splitter/6(Ltail) -> [Ltail]
  Mid-Range Component Splitter/7(Rimp) -> [Rimp]
  Mid-Range Component Splitter/8(Rtail) -> [Rtail]
  BS O/P/1 -> Discrete Surround Component Splitter/1(Discrete Surround Inputs)
  Discrete Surround Component Splitter/2(Lsi) -> [Lsi]
  Discrete Surround Component Splitter/1(Ci) -> [Ci]
  Discrete Surround Component Splitter/3(Rsi) -> [Rsi]
  [Lsi] -> Matrix Concatenate/8, Matrix Concatenate3/6
  [Rsi] -> Matrix Concatenate2/8, Matrix Concatenate5/6
  [Ci] -> Matrix Concatenate5/7, Matrix Concatenate2/9
  [Ci] -> Matrix Concatenate/9

== system MedusaPremix/Premix51WithMonoSurround/Merge NTF_done ==
  SLC_NTF_done_Left : Inport
  SLC_NTF_done_CS : Inport  Port=2
  SLC_NTF_done_Right : Inport  Port=3
  Trigger : TriggerPort  TriggerType=function-call  VariantControl=Variant  PortDimensions=1
  AND : Logic  Inputs=3  IconShape=distinctive  AllPortsSameDT=off  OutDataTypeStr=boolean
  SLC_NTF_done : Outport  VectorParamsAs1DForOutWhenUnconnected=off
  wires:
  SLC_NTF_done_Right/1 -> AND/1
  SLC_NTF_done_CS/1 -> AND/2
  SLC_NTF_done_Left/1 -> AND/3
  AND/1 -> SLC_NTF_done/1

== system MedusaPremix/Premix51WithMonoSurround/SLC Tuning ==
  Detent Level CS : Subsystem  Description="This is the premix (scalar mixing) matrix for the detent (default) level of \"surroundiness\"."
  Detent Level Left : Subsystem  Description="This is the premix (scalar mixing) matrix for the detent (default) level of \"surroundiness\"."
  Detent Level Right : Subsystem  Description="This is the premix (scalar mixing) matrix for the detent (default) level of \"surroundiness\"."
  Interpolation Method : Subsystem  Description=|
      | This controls the method used to interpolate premix coefficient matrix as the surround knob is adjusted.
      | - 0 for linear interpolation (default)
      | - 1 for db-linear interpolation
  Max Level CS : Subsystem  Description="This is the premix (scalar mixing) matrix for the maximum level of \"surroundiness\"."
  Max Level Left : Subsystem  Description="This is the premix (scalar mixing) matrix for the maximum level of \"surroundiness\"."
  Max Level Right : Subsystem  Description="This is the premix (scalar mixing) matrix for the maximum level of \"surroundiness\"."
  Min Level CS : Subsystem  Description="This is the premix (scalar mixing) matrix for the minimum level of \"surroundiness\" i.e. steroe case."
  Min Level Left : Subsystem  Description="This is the premix (scalar mixing) matrix for the minimum level of \"surroundiness\" i.e. steroe case."
  Min Level Right : Subsystem  Description="This is the premix (scalar mixing) matrix for the minimum level of \"surroundiness\" i.e. steroe case."
  Bus Element Out : Outport  VectorParamsAs1DForOutWhenUnconnected=off  PortName=SLC Tune Out  Element=Interpolation Method
  Bus Element Out1 : Outport  VectorParamsAs1DForOutWhenUnconnected=off  PortName=SLC Tune Out  Element=Min Level Left
  Bus Element Out2 : Outport  VectorParamsAs1DForOutWhenUnconnected=off  PortName=SLC Tune Out  Element=Detent Level Left
  Bus Element Out3 : Outport  VectorParamsAs1DForOutWhenUnconnected=off  PortName=SLC Tune Out  Element=Max Level Left
  Bus Element Out4 : Outport  VectorParamsAs1DForOutWhenUnconnected=off  PortName=SLC Tune Out  Element=Min Level CS
  Bus Element Out5 : Outport  VectorParamsAs1DForOutWhenUnconnected=off  PortName=SLC Tune Out  Element=Detent Level CS
  Bus Element Out6 : Outport  VectorParamsAs1DForOutWhenUnconnected=off  PortName=SLC Tune Out  Element=Max Level CS
  Bus Element Out7 : Outport  VectorParamsAs1DForOutWhenUnconnected=off  PortName=SLC Tune Out  Element=Min Level Right
  Bus Element Out8 : Outport  VectorParamsAs1DForOutWhenUnconnected=off  PortName=SLC Tune Out  Element=Detent Level Right
  Bus Element Out9 : Outport  VectorParamsAs1DForOutWhenUnconnected=off  PortName=SLC Tune Out  Element=Max Level Right
  wires:
  Interpolation Method/1(Out1) -> Bus Element Out/1
  Min Level Left/1(Out1) -> Bus Element Out1/1
  Detent Level Left/1(Out1) -> Bus Element Out2/1
  Max Level Left/1(Out1) -> Bus Element Out3/1
  Max Level CS/1(Out1) -> Bus Element Out6/1
  Min Level CS/1(Out1) -> Bus Element Out4/1
  Detent Level CS/1(Out1) -> Bus Element Out5/1
  Detent Level Right/1(Out1) -> Bus Element Out8/1
  Max Level Right/1(Out1) -> Bus Element Out9/1
  Min Level Right/1(Out1) -> Bus Element Out7/1

== system MedusaPremix/Premix51WithMonoSurroundAndCae/CS Processing ==
  COut : Inport
  ChanIn : Inport  Port=2
  MixCoeff : Inport  Port=3
  Constant : Constant  Value=MedusaPremixConfig.NumSurroundOut  SampleTime=-1
  Mono-Surround : Subsystem
  Selective Concatenation : MATLAB Function  TreatAsAtomicUnit=on
  CSOut : Outport  VectorParamsAs1DForOutWhenUnconnected=off
  wires:
  ChanIn/1 -> Mono-Surround/1(ChanIn)
  Mono-Surround/1(S) -> Selective Concatenation/2(S)
  COut/1 -> Selective Concatenation/1(COut)
  MixCoeff/1 -> Mono-Surround/2(MixCoeff)
  Selective Concatenation/1(CSOut) -> CSOut/1
  Constant/1 -> Mono-Surround/Enable
